simulink model "y103"  (R2019b)
settings: Solver=ode23tb  StartTime=0.0  StopTime=1  MaxStep=1e-4  RelTol=1e-3
undefined symbols (not defined in the file or in its folder): i
libraries: powerlib x9, simulink x1
settings Model: Creator=80573  LastModifiedBy=Inspiron
settings DataIOCC: ReturnWorkspaceOutputs=off
settings DebuggingCC: ArithmeticOperatorsInVariantConditions=warning
settings SFSimCC: SimUseLocalCustomCode=off  CustomCodeUndefinedFunction=UseInterfaceOnly
settings RTWCC: RTWUseLocalCustomCode=off

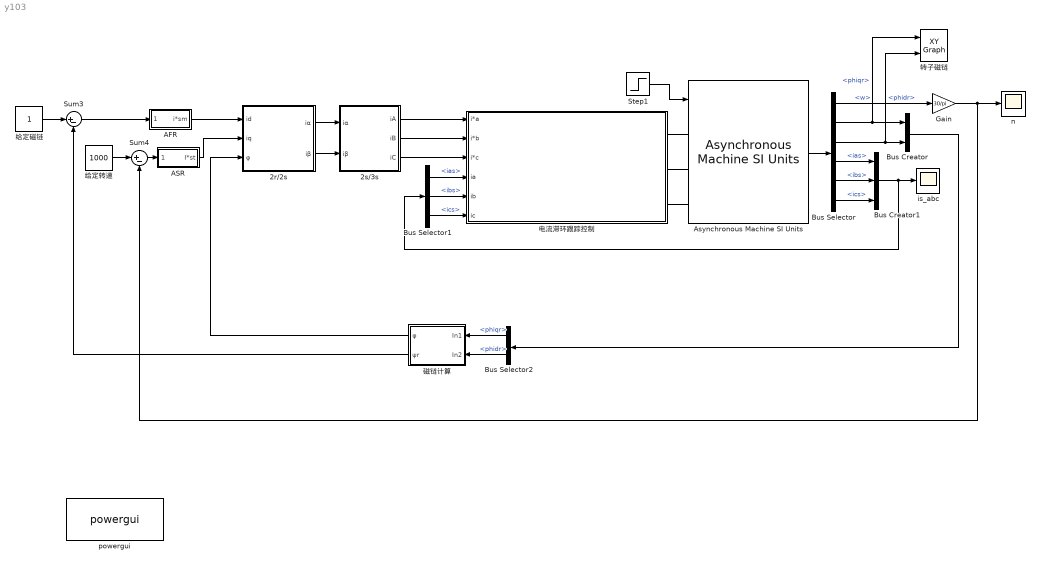
== system y103 ==
  2r/2s : Subsystem
  2s/3s : Subsystem
  AFR : Subsystem
  ASR : Subsystem
  Asynchronous Machine SI Units : powerlib/Machines/Asynchronous Machine SI Units  RotorType=Squirrel-cage  PresetModel=No  MechanicalLoad=Torque Tm  ShowDetailedParameters=on  ReferenceFrame=Stationary  Units=SI  MeasurementBus=on  NominalParameters=[2200 380 50]  Stator=[0.435 0.002]  Rotor=[0.816 0.002]  Cage1=[0.4155 0.002066]  Cage2=[0.4168 0.0003495]  Lm=0.069  Mechanical=[0.19 0 2]  PolePairs=2  InitialConditions=[1 0 0 0 0 0 0 0]  SimulateSaturation=off  Saturation=[14.03593122, 27.81365428, 53.79336849, 72.68890987, 97.98006896, 148.6815601, 215.7428561, 302.9841135, 428.7778367 ; 230, 322, 414, 460, 506, 552, 598, 644, 690]  LoadFlowParameters=1492000  TsPowergui=0  TsBlock=-1  IterativeModel=Trapezoidal non iterative  IterativeDiscreteModel=Trapezoidal non iterative  Pmec=1.492e+006
      settings: SourceProductName=Simscape Electrical
  Bus Creator : BusCreator  Inputs=2
  Bus Creator1 : BusCreator  Inputs=3
  Bus Selector : BusSelector  OutputSignals=w,phiqr,phidr,ias,ibs,ics
  Bus Selector1 : BusSelector  OutputSignals=ias,ibs,ics
  Bus Selector2 : BusSelector  OutputSignals=phiqr,phidr
  Gain : Gain  Gain=30/pi
  Step1 : Step  Time=0.6  After=55  SampleTime=0
  Sum3 : Sum  Inputs=|+-
  Sum4 : Sum  Inputs=|+-
  is_abc : Scope
  n : Scope
  powergui : powerlib/powergui  SimulationMode=Discrete  SampleTime=0.00001  frequency=50  Iterations=50  frequencyindice=50  Pbase=100e6  ErrMax=1e-4  UnitsV=kV  UnitsW=MW  buscounter=0  FunctionMessages=off  echomessages=off  EnableUseOfTLC=off  CurrentSourceSwitches=off  DisableSnubberDevices=off  DisableRonSwitches=off  DisableVfSwitches=off  DisplayEquations=off  AutomaticDiscreteSolvers=off  SolverType=Tustin/Backward Euler (TBE)  Interpol=off  ExternalGateDelay=off  methode=off  Ts=100  x0status=zero  SPID=on  SwTol=0  HookPort=off  NonlinearTolerance=1e-4  nMaxIteration=100  ContinueOnMaxIteration=off  RestoreLinks=warning  ResistiveCurrentMeasurement=off  Frange=[0:2:500]  Ylog=off  Xlog=on  ShowGrid=off  save=off  variable=ZData  structure=0  ZoomFFT=on  StartTime=0.0  cycles=1  DisplayStyle=1  fundamental=60  FreqAxis=off  MaxFrequency=1000  frequencyindicesteady=1  RmsSteady=1  display=off
      settings: SourceProductName=Simscape Electrical
  电流滞环跟踪控制 : Subsystem
  磁链计算 : Subsystem
  给定磁链 : Constant
  给定转速 : Constant  Value=1000
  转子磁链 : simulink/Sinks/XY Graph  xmin=-1  xmax=1  ymin=-1  ymax=1  st=-1
  wires:
  Step1/1 -> Asynchronous Machine SI Units/1
  Sum3/1 -> AFR/1(" ")
  Sum4/1 -> ASR/1("  ")
  给定磁链/1 -> Sum3/1
  AFR/1(i*sm) -> 2r/2s/1(id)
  Bus Selector/4 -> Bus Creator1/1  "<ias>"
  Bus Selector/6 -> Bus Creator1/3  "<ics>"
  Bus Selector/2 -> Bus Creator/1, 转子磁链/1  "<phiqr>"
  Bus Selector/5 -> Bus Creator1/2  "<ibs>"
  Bus Selector/1 -> Gain/1  "<w>"
  Bus Creator1/1 -> Bus Selector1/1, is_abc/1
  Asynchronous Machine SI Units/1 -> Bus Selector/1
  给定转速/1 -> Sum4/1
  Gain/1 -> n/1, Sum4/2
  2r/2s/1(iα) -> 2s/3s/1(iα)
  2r/2s/2(iβ) -> 2s/3s/2(iβ)
  2s/3s/1(iA) -> 电流滞环跟踪控制/1(i*a)
  2s/3s/2(iB) -> 电流滞环跟踪控制/2(i*b)
  2s/3s/3(iC) -> 电流滞环跟踪控制/3(i*c)
  Bus Selector1/1 -> 电流滞环跟踪控制/4(ia)  "<ias>"
  Bus Selector1/2 -> 电流滞环跟踪控制/5(ib)  "<ibs>"
  Bus Selector1/3 -> 电流滞环跟踪控制/6(ic)  "<ics>"
  ASR/1(I*st) -> 2r/2s/2(iq)
  磁链计算/2(ψr) -> Sum3/2
  磁链计算/1(φ) -> 2r/2s/3(φ)
  Bus Selector/3 -> Bus Creator/2, 转子磁链/2  "<phidr>"
  Bus Creator/1 -> Bus Selector2/1
  Bus Selector2/1 -> 磁链计算/1(In1)  "<phiqr>"
  Bus Selector2/2 -> 磁链计算/2(In2)  "<phidr>"
  connections:
  电流滞环跟踪控制/RConn1 -- Asynchronous Machine SI Units/LConn1
  电流滞环跟踪控制/RConn2 -- Asynchronous Machine SI Units/LConn2
  电流滞环跟踪控制/RConn3 -- Asynchronous Machine SI Units/LConn3

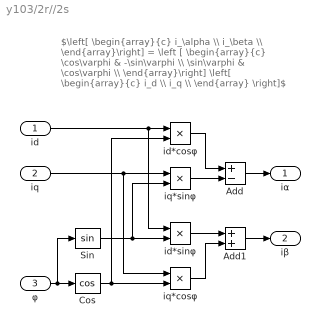
== system y103/2r//2s ==
  note: $\left[ \begin{array}{c} i_\alpha \\ i_\beta \\ \end{array}\right] = \left [ \begin{array}{c} \cos\varphi & -\sin\varphi \\ \sin\varphi & \cos\varphi \\ \end{array}\right] \left[ \begin{array}{c} i_d \\ i_q \\ \end{array} \right]$
  id : Inport
  iq : Inport  Port=2
  φ : Inport  Port=3
  Add : Sum  Inputs=+-
  Add1 : Sum
  Cos : Trigonometry  Operator=cos
  Sin : Trigonometry
  id*cosφ : Product
  id*sinφ : Product
  iq*cosφ : Product
  iq*sinφ : Product
  iα : Outport
  iβ : Outport  Port=2
  wires:
  Cos/1 -> iq*cosφ/2, id*cosφ/2
  iq*cosφ/1 -> Add1/2
  Sin/1 -> id*sinφ/2, iq*sinφ/2
  id/1 -> id*cosφ/1, id*sinφ/1
  id*sinφ/1 -> Add1/1
  iq*sinφ/1 -> Add/2
  iq/1 -> iq*sinφ/1, iq*cosφ/1
  φ/1 -> Sin/1, Cos/1
  Add/1 -> iα/1
  id*cosφ/1 -> Add/1
  Add1/1 -> iβ/1

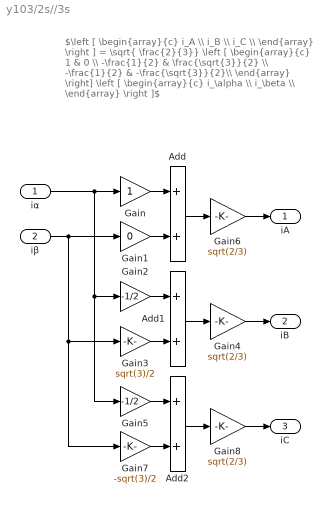
== system y103/2s//3s ==
  note: $\left [ \begin{array}{c} i_A \\ i_B \\ i_C \\ \end{array} \right ] = \sqrt{ \frac{2}{3}} \left [ \begin{array}{c} 1 & 0 \\ -\frac{1}{2} & \frac{\sqrt{3}}{2} \\ -\frac{1}{2} & -\frac{\sqrt{3}}{2}\\ \end{array} \right] \left [ \begin{array}{c} i_\alpha \\ i_\beta \\ \end{array} \right ]$
  iα : Inport
  iβ : Inport  Port=2
  Add : Sum  Inputs=2
  Add1 : Sum  Inputs=2
  Add2 : Sum  Inputs=2
  Gain : Gain
  Gain1 : Gain  Gain=0
  Gain2 : Gain  Gain=-1/2
  Gain3 : Gain  Gain=sqrt(3)/2
  Gain4 : Gain  Gain=sqrt(2/3)
  Gain5 : Gain  Gain=-1/2
  Gain6 : Gain  Gain=sqrt(2/3)
  Gain7 : Gain  Gain=-sqrt(3)/2
  Gain8 : Gain  Gain=sqrt(2/3)
  iA : Outport
  iB : Outport  Port=2
  iC : Outport  Port=3
  wires:
  Gain/1 -> Add/1
  iβ/1 -> Gain7/1, Gain3/1, Gain1/1
  Add/1 -> Gain6/1
  Gain1/1 -> Add/2
  iα/1 -> Gain5/1, Gain2/1, Gain/1
  Gain4/1 -> iB/1
  Gain6/1 -> iA/1
  Gain2/1 -> Add1/1
  Gain3/1 -> Add1/2
  Add1/1 -> Gain4/1
  Gain5/1 -> Add2/1
  Gain7/1 -> Add2/2
  Gain8/1 -> iC/1
  Add2/1 -> Gain8/1

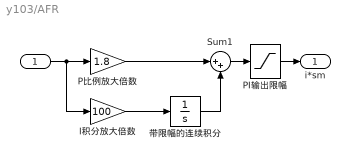
== system y103/AFR ==
  " " : Inport
  I积分放大倍数 : Gain  Gain=100
  PI输出限幅 : Saturate  UpperLimit=13  LowerLimit=-13
  P比例放大倍数 : Gain  Gain=1.8
  Sum1 : Sum  Inputs=|++
  带限幅的连续积分 : Integrator  LimitOutput=on  UpperSaturationLimit=15  LowerSaturationLimit=-15
  i*sm : Outport  VectorParamsAs1DForOutWhenUnconnected=off
  wires:
  Sum1/1 -> PI输出限幅/1
  PI输出限幅/1 -> i*sm/1
  I积分放大倍数/1 -> 带限幅的连续积分/1
  P比例放大倍数/1 -> Sum1/1
  带限幅的连续积分/1 -> Sum1/2
  " "/1 -> I积分放大倍数/1, P比例放大倍数/1

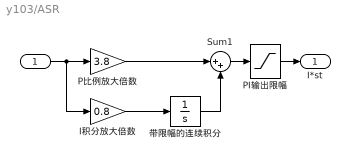
== system y103/ASR ==
  "  " : Inport
  I积分放大倍数 : Gain  Gain=0.8
  PI输出限幅 : Saturate  UpperLimit=75  LowerLimit=-75
  P比例放大倍数 : Gain  Gain=3.8
  Sum1 : Sum  Inputs=|++
  带限幅的连续积分 : Integrator  LimitOutput=on  UpperSaturationLimit=80  LowerSaturationLimit=-80
  I*st : Outport  VectorParamsAs1DForOutWhenUnconnected=off
  wires:
  Sum1/1 -> PI输出限幅/1
  PI输出限幅/1 -> I*st/1
  P比例放大倍数/1 -> Sum1/1
  I积分放大倍数/1 -> 带限幅的连续积分/1
  带限幅的连续积分/1 -> Sum1/2
  "  "/1 -> I积分放大倍数/1, P比例放大倍数/1

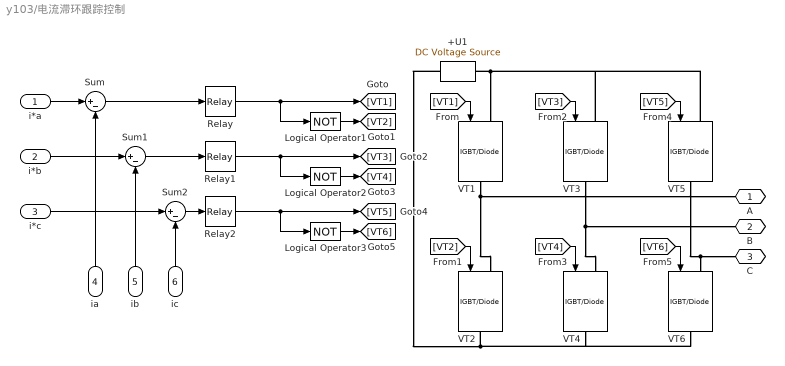
== system y103/电流滞环跟踪控制 ==
  i*a : Inport
  i*b : Inport  Port=2
  i*c : Inport  Port=3
  ia : Inport  Port=4
  ib : Inport  Port=5
  ic : Inport  Port=6
  +U1 : powerlib/Electrical Sources/DC Voltage Source  Amplitude=510  Measurements=None
      settings: SourceProductName=Simscape Electrical
  Logical Operator1 : Logic  Operator=NOT  AllPortsSameDT=off  OutDataTypeStr=boolean
  Logical Operator2 : Logic  Operator=NOT  AllPortsSameDT=off  OutDataTypeStr=boolean
  Logical Operator3 : Logic  Operator=NOT  AllPortsSameDT=off  OutDataTypeStr=boolean
  Relay : Relay  OnSwitchValue=0.2  OffSwitchValue=-0.2
  Relay1 : Relay  OnSwitchValue=0.2  OffSwitchValue=-0.2
  Relay2 : Relay  OnSwitchValue=0.2  OffSwitchValue=-0.2
  Sum : Sum  Inputs=|+-
  Sum1 : Sum  Inputs=|+-
  Sum2 : Sum  Inputs=|+-
  VT{1..6} (6 alike) : powerlib/Power Electronics/IGBT//Diode  Ron=1e-3  Rs=1e5  Cs=inf  Measurements=off
      settings: SourceProductName=Simscape Electrical
  A : PMIOPort  Side=Right
  B : PMIOPort  Port=2  Side=Right
  C : PMIOPort  Port=3  Side=Right
  wires:
  [VT3] -> VT3/1
  Relay/1 -> Logical Operator1/1, [VT1]
  [VT4] -> VT4/1
  Sum2/1 -> Relay2/1
  Relay1/1 -> Logical Operator2/1, [VT3]
  ic/1 -> Sum2/2
  Sum/1 -> Relay/1
  Sum1/1 -> Relay1/1
  [VT5] -> VT5/1
  Logical Operator3/1 -> [VT6]
  Relay2/1 -> Logical Operator3/1, [VT5]
  i*c/1 -> Sum2/1
  ia/1 -> Sum/2
  Logical Operator2/1 -> [VT4]
  [VT6] -> VT6/1
  [VT2] -> VT2/1
  Logical Operator1/1 -> [VT2]
  [VT1] -> VT1/1
  ib/1 -> Sum1/2
  i*a/1 -> Sum/1
  i*b/1 -> Sum1/1
  connections:
  +U1/RConn1 -- VT3/LConn1 -- VT5/LConn1 -- VT1/LConn1
  VT6/RConn1 -- VT4/RConn1 -- +U1/LConn1 -- VT2/RConn1
  VT5/RConn1 -- C/RConn1 -- VT6/LConn1
  VT3/RConn1 -- VT4/LConn1 -- B/RConn1
  VT1/RConn1 -- VT2/LConn1 -- A/RConn1

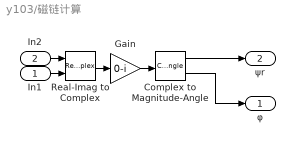
== system y103/磁链计算 ==
  In1 : Inport
  In2 : Inport  Port=2
  Complex to Magnitude-Angle : ComplexToMagnitudeAngle
  Gain : Gain  Gain=0-i
  Real-Imag to Complex : RealImagToComplex
  φ : Outport
  ψr : Outport  Port=2
  wires:
  Complex to Magnitude-Angle/1 -> ψr/1
  Complex to Magnitude-Angle/2 -> φ/1
  Gain/1 -> Complex to Magnitude-Angle/1
  Real-Imag to Complex/1 -> Gain/1
  In1/1 -> Real-Imag to Complex/2
  In2/1 -> Real-Imag to Complex/1
